simulink model "IfActionSubsystem_SpeedConyrol"  (R2021a)
settings: Solver=VariableStepAuto  StartTime=0.0  StopTime=10.0  RelTol=1e-3
libraries: simulink x1
settings Model: Creator=lenovo  LastModifiedBy=lenovo

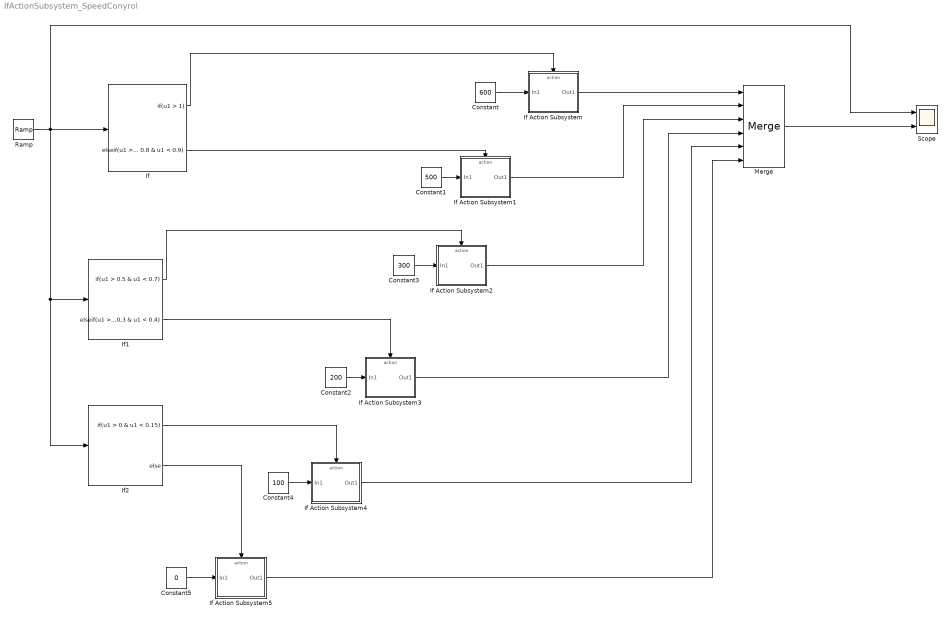
== system IfActionSubsystem_SpeedConyrol ==
  Constant : Constant  Value=600
  Constant1 : Constant  Value=500
  Constant2 : Constant  Value=200
  Constant3 : Constant  Value=300
  Constant4 : Constant  Value=100
  Constant5 : Constant  Value=0
  If : If  IfExpression=u1 > 1  ElseIfExpressions=u1 > 0.8 & u1 < 0.9  ShowElse=off
  If Action Subsystem : Subsystem  TreatAsAtomicUnit=on
  If Action Subsystem1 : Subsystem  TreatAsAtomicUnit=on
  If Action Subsystem2 : Subsystem  TreatAsAtomicUnit=on
  If Action Subsystem3 : Subsystem  TreatAsAtomicUnit=on
  If Action Subsystem4 : Subsystem  TreatAsAtomicUnit=on
  If Action Subsystem5 : Subsystem  TreatAsAtomicUnit=on
  If1 : If  IfExpression=u1 > 0.5 & u1 < 0.7  ElseIfExpressions=u1 > 0.3 & u1 < 0.4  ShowElse=off
  If2 : If  IfExpression=u1 > 0 & u1 < 0.15
  Merge : Merge  Inputs=6
  Ramp : simulink/Sources/Ramp  slope=1  start=0  InitialOutput=0
  Scope : Scope  NumInputPorts=2
  wires:
  If Action Subsystem1/1(Out1) -> Merge/2
  If Action Subsystem/1(Out1) -> Merge/1
  If Action Subsystem2/1(Out1) -> Merge/3
  Merge/1 -> Scope/2
  Constant3/1 -> If Action Subsystem2/1(In1)
  Constant/1 -> If Action Subsystem/1(In1)
  Constant1/1 -> If Action Subsystem1/1(In1)
  Ramp/1 -> If2/1, If1/1, Scope/1, If/1
  If1/1 -> If Action Subsystem2/Action
  If/1 -> If Action Subsystem/Action
  If/2 -> If Action Subsystem1/Action
  Constant2/1 -> If Action Subsystem3/1(In1)
  If1/2 -> If Action Subsystem3/Action
  Constant4/1 -> If Action Subsystem4/1(In1)
  Constant5/1 -> If Action Subsystem5/1(In1)
  If2/1 -> If Action Subsystem4/Action
  If2/2 -> If Action Subsystem5/Action
  If Action Subsystem3/1(Out1) -> Merge/4
  If Action Subsystem4/1(Out1) -> Merge/5
  If Action Subsystem5/1(Out1) -> Merge/6

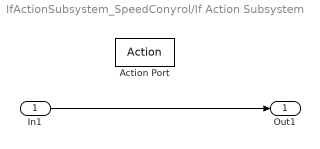
== system IfActionSubsystem_SpeedConyrol/If Action Subsystem ==
  In1 : Inport
  Action Port : ActionPort  ActionPortLabel=if(u1 > 1)
  Out1 : Outport
  wires:
  In1/1 -> Out1/1

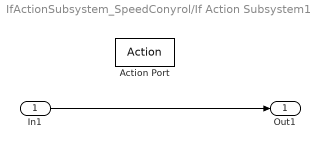
== system IfActionSubsystem_SpeedConyrol/If Action Subsystem1 ==
  In1 : Inport
  Action Port : ActionPort  ActionPortLabel=elseif(u1 > 0.8 & u1 < 0.9)
  Out1 : Outport
  wires:
  In1/1 -> Out1/1

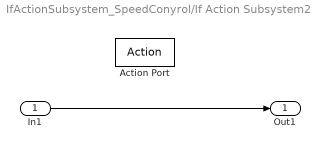
== system IfActionSubsystem_SpeedConyrol/If Action Subsystem2 ==
  In1 : Inport
  Action Port : ActionPort  ActionPortLabel=if(u1 > 0.5 & u1 < 0.7)
  Out1 : Outport
  wires:
  In1/1 -> Out1/1

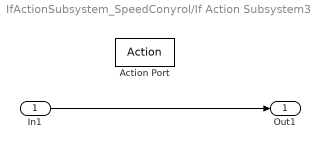
== system IfActionSubsystem_SpeedConyrol/If Action Subsystem3 ==
  In1 : Inport
  Action Port : ActionPort  ActionPortLabel=elseif(u1 > 0.3 & u1 < 0.4)
  Out1 : Outport
  wires:
  In1/1 -> Out1/1

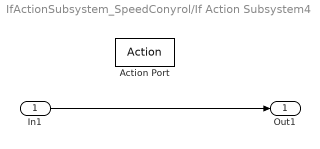
== system IfActionSubsystem_SpeedConyrol/If Action Subsystem4 ==
  In1 : Inport
  Action Port : ActionPort  ActionPortLabel=if(u1 > 0 & u1 < 0.15)
  Out1 : Outport
  wires:
  In1/1 -> Out1/1

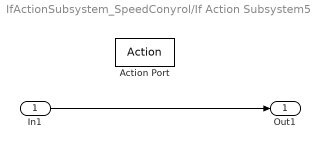
== system IfActionSubsystem_SpeedConyrol/If Action Subsystem5 ==
  In1 : Inport
  Action Port : ActionPort  ActionPortLabel=else
  Out1 : Outport
  wires:
  In1/1 -> Out1/1
